simulink subsystem "Subsystem_PieroControladoV"  (R2023b)
settings: Solver=VariableStepAuto  StartTime=0.0  StopTime=10.0  RelTol=1e-3
settings Model: Creator=Alberto  LastModifiedBy=Alberto

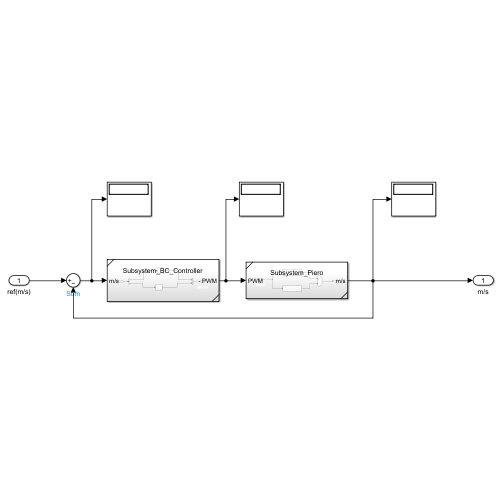
[thumbnail: Simulink's stored preview of the top-level diagram]
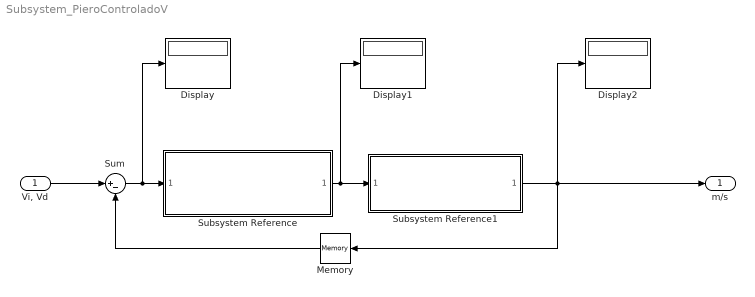
== system Subsystem_PieroControladoV ==
  "Vi, Vd" : Inport
  Display : Display
  Display1 : Display
  Display2 : Display
  Memory : Memory
  Subsystem Reference : Subsystem  ReferencedSubsystem=Subsystem_BC_Controller
  Subsystem Reference1 : Subsystem  ReferencedSubsystem=Subsystem_Piero
  Sum : Sum  Inputs=|+-
  m/s : Outport
  wires:
  Subsystem Reference/1 -> Display1/1, Subsystem Reference1/1
  Subsystem Reference1/1 -> m/s/1, Display2/1, Memory/1
  "Vi, Vd"/1 -> Sum/1
  Sum/1 -> Display/1, Subsystem Reference/1
  Memory/1 -> Sum/2
